simulink model "mcb_microchip_pmsm_foc_sensorless_dsPIC33EP256MC506"  (R2024b)
settings: Solver=FixedStepDiscrete  StartTime=0.0  StopTime=10  FixedStep=Ts  RelTol=1e-3  EnableMultiTasking=on
InitFcn:
  | mcb_microchip_pmsm_foc_sensorless_dsPIC33_data;
undefined symbols (not defined in the file): A4, C5, D8, F1, inverter, P20, P53, P97, PI_params, Pin, pmsm, PU_System, PWM_frequency, PWMmax, Speed_openLoop_PU, Ts, Ts_speed
libraries: MCHP_Blockset x16, mcbcontrolslib x10, simulink x9, slpidlib x3, mcbpositiondecoderlib x2, mcbplantlib x1, autolibpmsmexterior x1
(part 2 of 3)

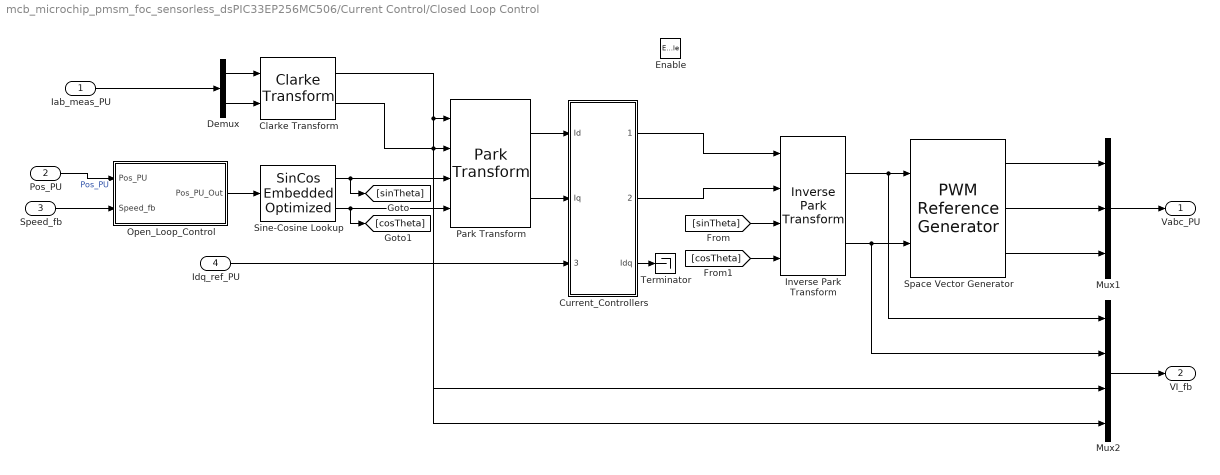
== system mcb_microchip_pmsm_foc_sensorless_dsPIC33EP256MC506/Current Control/Closed Loop Control ==
  Iab_meas_PU : Inport
  Pos_PU : Inport  Port=2
  Speed_fb : Inport  Port=3
  Idq_ref_PU : Inport  Port=4
  Enable : EnablePort
  Clarke Transform : mcbcontrolslib/Clarke Transform  VariantControl=Variant2  PhaseInput=Two inputs  EnPowerInv=off
  Current_Controllers : Subsystem
  Demux : Demux  Outputs=2
  Inverse Park Transform : mcbcontrolslib/Inverse Park Transform  PhaseInput=Two inputs  AxisAlignment=D-axis  ThetaInput=Sine and Cosine electrical position  AngleInput=Per-unit  N_points=1024
  Mux1 : Mux  Inputs=3
  Mux2 : Mux
  Open_Loop_Control : Subsystem
  Park Transform : mcbcontrolslib/Park Transform  PhaseInput=Two inputs  AxisAlignment=D-axis  ThetaInput=Sine and Cosine electrical position  AngleInput=Per-unit  N_points=1024
  Sine-Cosine Lookup : mcbcontrolslib/SinCos Embedded Optimized  LabelModeActiveChoice=MCB_Sin  OptforProc=off  ApproximationMethod=None  UserApproxMethod=Lookup  ApproxStatus=None  InterpMethod=Linear point-slope  NumberOfDataPoints=16  NumberOfIterations=11  RemoveProtectionAgainstOutOfRangeInput=off  TableDataTypeStr=Inherit: Inherit via input  AngleInput=Per-unit  ThetaDataType=single  N_points=1024  DatatypeInput=Inherit from input  Datatype=Inherit: Same as input
  Space Vector Generator : mcbcontrolslib/PWM Reference Generator  inSignal=Valphabeta  modType=SVM: space vector modulation
  Terminator : Terminator
  Vabc_PU : Outport  OutputWhenDisabled=reset  InitialOutput=[0 0 0]  VectorParamsAs1DForOutWhenUnconnected=off
  VI_fb : Outport  Port=2  OutputWhenDisabled=reset  InitialOutput=[0 0 0 0]  VectorParamsAs1DForOutWhenUnconnected=off
  wires:
  Current_Controllers/1(Vd_ref) -> Inverse Park Transform/1
  [sinTheta] -> Inverse Park Transform/3
  Sine-Cosine Lookup/1 -> [sinTheta], Park Transform/3
  Space Vector Generator/1 -> Mux1/1
  Space Vector Generator/3 -> Mux1/3
  Sine-Cosine Lookup/2 -> Park Transform/4, [cosTheta]
  Space Vector Generator/2 -> Mux1/2
  Idq_ref_PU/1 -> Current_Controllers/3(Idq_ref_PU)
  Iab_meas_PU/1 -> Demux/1
  Demux/1 -> Clarke Transform/1
  Demux/2 -> Clarke Transform/2
  Park Transform/2 -> Current_Controllers/2(Iq)
  [cosTheta] -> Inverse Park Transform/4
  Current_Controllers/2(Vq_ref) -> Inverse Park Transform/2
  Mux1/1 -> Vabc_PU/1
  Speed_fb/1 -> Open_Loop_Control/2(Speed_fb)
  Current_Controllers/3(Idq) -> Terminator/1
  Park Transform/1 -> Current_Controllers/1(Id)
  Pos_PU/1 -> Open_Loop_Control/1(Pos_PU)  "Pos_PU"
  Open_Loop_Control/1(Pos_PU_Out) -> Sine-Cosine Lookup/1
  Mux2/1 -> VI_fb/1
  Inverse Park Transform/1 -> Mux2/1, Space Vector Generator/1
  Clarke Transform/2 -> Mux2/4, Park Transform/2
  Inverse Park Transform/2 -> Space Vector Generator/2, Mux2/2
  Clarke Transform/1 -> Mux2/3, Park Transform/1

== system mcb_microchip_pmsm_foc_sensorless_dsPIC33EP256MC506/Current Control/Input Scaling ==
  Iab_PU_In : Inport
  Iab_PU_Sim : Inport  Port=2
  VI_fb : Inport  Port=3
  DC component removal : Subsystem
  Sensorless : Subsystem
  Variant Source : VariantSource
  Iab_PU : Outport
  Pos_PU : Outport  Port=2
  Speed_meas_PU : Outport  Port=3
  tag scope: Speed=global
  wires:
  Iab_PU_Sim/1 -> Variant Source/2
  Variant Source/1 -> Iab_PU/1
  DC component removal/1(SigOUT) -> Sensorless/1(VI_fb)
  VI_fb/1 -> DC component removal/1(SigIN)  "Pos"
  Sensorless/2(Theta) -> Pos_PU/1  "Pos"
  Sensorless/1(Speed_meas_PU) -> [Speed], Speed_meas_PU/1
  Iab_PU_In/1 -> Variant Source/1

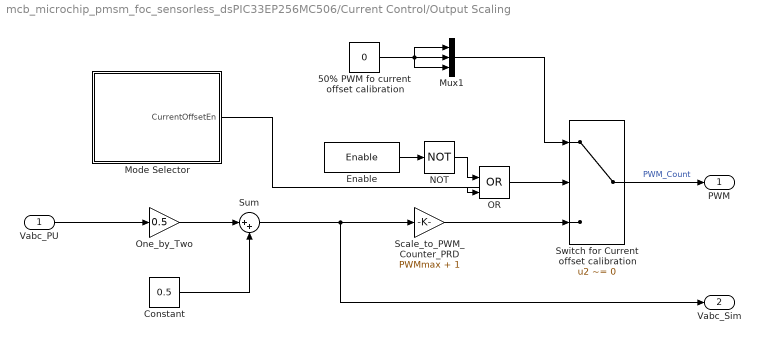
== system mcb_microchip_pmsm_foc_sensorless_dsPIC33EP256MC506/Current Control/Output Scaling ==
  Vabc_PU : Inport
  50% PWM fo current offset calibration : Constant  Value=0  OutDataTypeStr=Inherit: Inherit via back propagation
  Constant : Constant  Value=0.5  OutDataTypeStr=dataType  SampleTime=-1
  Enable : DataStoreRead  DataStoreName=Enable  IndexOptions=Index vector (dialog)  Indices=1  OutputSizes=1
  Mode Selector : Subsystem
  Mux1 : Mux  Inputs=3
  NOT : Logic  Operator=NOT  IconShape=distinctive  AllPortsSameDT=off  OutDataTypeStr=boolean
  OR : Logic  Operator=OR  IconShape=distinctive  AllPortsSameDT=off  OutDataTypeStr=boolean
  One_by_Two : Gain  Gain=0.5  RndMeth=Simplest  OutDataTypeStr=Inherit: Same as input
  Scale_to_PWM_Counter_PRD : Gain  Gain=PWMmax + 1  OutDataTypeStr=uint16  RndMeth=Simplest
  Sum : Sum  Inputs=|++
  Switch for Current offset calibration : Switch  Criteria=u2 ~= 0  Threshold=250  SaturateOnIntegerOverflow=off  InputSameDT=off
  PWM : Outport
  Vabc_Sim : Outport  Port=2
  wires:
  Constant/1 -> Sum/2
  One_by_Two/1 -> Sum/1
  Vabc_PU/1 -> One_by_Two/1
  Mux1/1 -> Switch for Current offset calibration/1
  50% PWM fo current offset calibration/1 -> Mux1/1, Mux1/3, Mux1/2
  Mode Selector/1(CurrentOffsetEn) -> OR/2
  OR/1 -> Switch for Current offset calibration/2
  Enable/1 -> NOT/1
  NOT/1 -> OR/1
  Scale_to_PWM_Counter_PRD/1 -> Switch for Current offset calibration/3
  Sum/1 -> Vabc_Sim/1, Scale_to_PWM_Counter_PRD/1
  Switch for Current offset calibration/1 -> PWM/1  "PWM_Count"

== system mcb_microchip_pmsm_foc_sensorless_dsPIC33EP256MC506/Current Control/PWM Driver ==
  PWM (abc) : Inport
  Dead time Compensation : Bias  Bias=round( (inverter.deadtime/Ts) *PWMmax )  SaturateOnIntegerOverflow=off
  Demux : Demux  Outputs=3
  PWM High Speed : MCHP_Blockset/PWM IO/PWM High Speed  pop1=[1]  chk1="[1  1  1  0  0]"  chkHL1="[1  1  1  1  1  1  1  1 ; 1  1  1  1  1  1  1  1]"  maxP1={ 'Ts','5e-05','5e-05','0.001','0.001','0.001','0.001','0.001';'0.001','0.001','1e-06','0.001','0.001','0.001','0.001','0.001'}  InitP2={ 'Ts','5e-05','5e-05','0.001','0.001','0.001','0.001','0.001';'0.001','0.001','0.001','0.001','0.001','0.001','0.001','0.001'}  chkP2="[0  0  0  1  1  1  1  1 ; 1  0  0  1  1  1  1  1]"  InitDC={ '4','4','4','50','50','50','50','50';'0.001','0.001','0.001','50','50','50','50','50'}  chkDC="[1  1  1  1  1  1  1  1 ; 0  0  0  1  1  1  1  1]"  InitPh={ '0','0','0','0.001','0.001','0.001','0.001','0.001';'0','0','0','0.001','0.001','0.001','0.001','0.001'}  chkPh="[0  0  0  1  1  1  1  1 ; 0  0  0  1  1  1  1  1]"  edSEvTrigx={ '0','-1','-1','-1','-1','-1','-1','-1'}  chkSEvTrigx="[0  0  0  1  1  1  1  1]"  popFlt="[2  2  2  1  1  1  1  1]"  popFltPin="[20  20  20   4   4   4   4   4]"  popFltPinRp="[1  1  1  1  1  1  1]"  popFltActivH="[2  2  2  1  1  1  1  1]"  popFltForceH="[2  2  2  2  2  2  2  2]"  popFltForceL="[1  1  1  1  1  1  1  1]"  chkFltBlkOut="[0  0  0  0  0  0  0  0]"  popIndepFaultMode="[1  1  1  1  1  1  1  1]"  popCurEnabled="[1  1  1  1  1  1  1  1]"  popCurPin="[4  31   4   4   4   4   4   4]"  popCurActiveH="[1  1  1  1  1  1  1  1]"  popCurForceH="[2  1  2  1  1  1  1  1]"  popCurForceL="[2  1  2  1  1  1  1  1]"  ChkCurBlkOut="[1  0  0  0  0  0  0  0]"  ChkCurBlkOutTime="[1  0  1  0  0  0  0  0]"  popBLANKSEL="[1  1  1  1  1  1  1  1]"  popBPHHBPHL="[1  1  1  1  1  1  1  1]"  popBPLHBPLL="[1  1  1  1  1  1  1  1]"  popFLTLEBEN_CLLEBEN="[1  1  1  1  1  1  1  1]"  popPHR_PHF="[2  1  1  1  1  1  1  1]"  popPLR_PLF="[3  1  1  1  1  1  1  1]"  edLEB={ '100e-9','50e-9','150e-9','50e-9','50e-9','50e-9','50e-9','50e-9'}  popDT="[1  1  1  3  3  3  3  3]"  edDTRx={ '0','0','0','1e-05','1e-05','1e-05','1e-05','1e-05'}  edAltDTRx={ 'inverter.deadtime','inverter.deadtime','inverter.deadtime','1e-05','1e-05','1e-05','1e-05','1e-05'}  S_INPUT="[5  5  5]"  S_INPUT_Size="[1  1  1]"  S_OUTPUT=[]  S_OUTPUT_Size=[]  S_DWORK_Type=[]  S_DWORK_Size=[]  ADC_VARTRIG={PWM Primary Special Event Trigger;6}  evalin_ws=PWMmax = 3499;PWM1max = 3499;PWM2max = 3499;PWM3max = 3499;  SampleTime=-1  ORDERING=None  MCHP_PORT={PWM1 Fault}{FLT32}4:0:B4;{PWM2 Fault}{FLT32}4:0:B4;{PWM3 Fault}{FLT32}4:0:B4;{PWM1H}{PWM1H}4:4:B14;{PWM1L}{PWM1L}4:4:B15;{PWM2H}{PWM2H}4:4:B12;{PWM2L}{PWM2L}4:4:B13;{PWM3H}{PWM3H}4:4:B10;{PWM3L}{PWM3L}4:4:B11;  MCHP_MASTERLINK=mcb_microchip_pmsm_foc_sensorless_dsPIC33EP256MC506/Hardware Init/Microchip Master  MCHP_VERSION=v3.38  Parameter50=0
      settings: SourceProductName=MPLAB Device Blocks for Simulink
  Saturation low side turn on errate workaround + errata for Phase shift (times 2) : Saturate  UpperLimit=PWMmax  LowerLimit=round( (inverter.deadtime/Ts) *PWMmax )* 2
  int to uint : DataTypeConversion  OutDataTypeStr=uint16  ConvertRealWorld=Stored Integer (SI)  SaturateOnIntegerOverflow=off  RndMeth=Floor
  wires:
  int to uint/1 -> Saturation low side turn on errate workaround + errata for Phase shift (times 2)/1
  Dead time Compensation/1 -> int to uint/1
  PWM (abc)/1 -> Dead time Compensation/1
  Saturation low side turn on errate workaround + errata for Phase shift (times 2)/1 -> Demux/1
  Demux/1 -> PWM High Speed/1
  Demux/2 -> PWM High Speed/2
  Demux/3 -> PWM High Speed/3

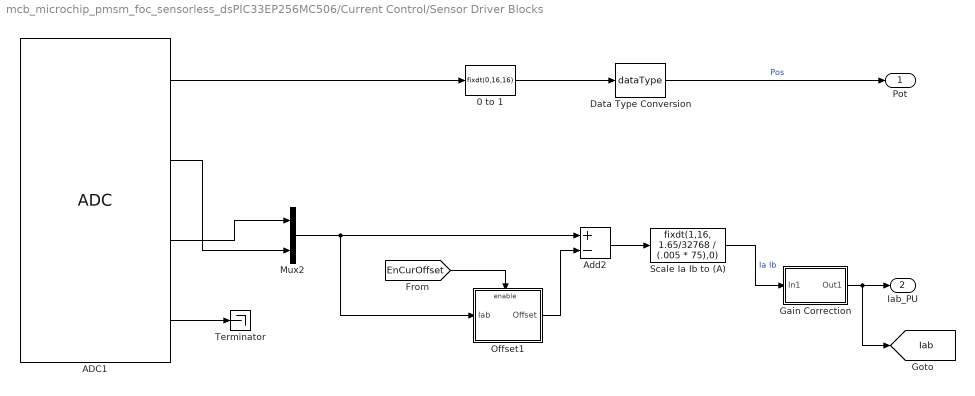
== system mcb_microchip_pmsm_foc_sensorless_dsPIC33EP256MC506/Current Control/Sensor Driver Blocks ==
  0 to 1 : DataTypeConversion  OutDataTypeStr=fixdt(0,16,16)  ConvertRealWorld=Stored Integer (SI)  SaturateOnIntegerOverflow=off  RndMeth=Floor
  ADC1 : MCHP_Blockset/Analog IO/ADC  Priority=5  ADC_REF=1  Mode=10 bits (allows exact simultaneous sampling)  FORM=dddd dddd dddd 0000 ==> Unsigned fractional  ADC_R="< 5    kOhm"  nSAMPLECHANNELS=CH0 : CH1 : CH2 : CH3  nSAMPLECHANNELS_12bits=CH0 only  SIMULTANEOUS=Simultaneously on all Channels  ADxCSS=[13]  MUXA_CH0N=off  MUXA_CH123_TXT=AN0 : AN1 : AN2  MUXB_CH0=AN13  MUXB_CH0N=on  MUXB_CH123_TXT=AN0 : AN1 : AN2  SequenceRepeat=1  SequenceTiming=are done as fast as possible ; triggered by user define source  SSRC_SSRCG_TXT=6  Update_BlockOutput=After each trig and conversion sequence  Trig_TimeStep=with each update of the ADC block output  ADC_DMA_CHANNEL=Use Interrupt instead of DMA  SampleTime=5e-05  Info=Total Time for Sample & Conversion : 4.4571e-06s including 3.4286e-07s (x 1) sample time.  MCHP_PORT={Analog Input 0}{AN0}15:2:A0;{Analog Input 1}{AN1}15:2:A1;{Analog Input 2}{AN2}15:2:B0;{Analog Input 13}{AN13}15:2:E13;  MCHP_MASTERLINK=mcb_microchip_pmsm_foc_sensorless_dsPIC33EP256MC506/Hardware Init/Microchip Master  ADC_TIMING=[4.4571428571428571832e-06]
      settings: SourceProductName=MPLAB Device Blocks for Simulink
  Add2 : Sum  Inputs=+-  OutDataTypeStr=int16  RndMeth=Zero
  Data Type Conversion : DataTypeConversion  OutDataTypeStr=dataType  RndMeth=Simplest  SaturateOnIntegerOverflow=off
  Gain Correction : Subsystem
  Mux2 : Mux  Inputs=2
  Offset1 : Subsystem
  Scale Ia Ib to (A) : DataTypeConversion  OutDataTypeStr=fixdt(1,16, 1.65/32768 / (.005 * 75),0)  ConvertRealWorld=Stored Integer (SI)  SaturateOnIntegerOverflow=off
  Terminator : Terminator
  Pot : Outport  VectorParamsAs1DForOutWhenUnconnected=off
  Iab_PU : Outport  Port=2  VectorParamsAs1DForOutWhenUnconnected=off
  tag scope: Iab=global
  wires:
  Mux2/1 -> Offset1/1(Iab), Add2/1
  0 to 1/1 -> Data Type Conversion/1
  [EnCurOffset] -> Offset1/Enable
  Data Type Conversion/1 -> Pot/1  "Pos"
  Add2/1 -> Scale Ia Ib to (A)/1
  ADC1/3 -> Mux2/1
  ADC1/1 -> 0 to 1/1
  Offset1/1(Offset) -> Add2/2
  ADC1/2 -> Mux2/2
  ADC1/4 -> Terminator/1
  Scale Ia Ib to (A)/1 -> Gain Correction/1(In1)  "Ia Ib"
  Gain Correction/1(Out1) -> [Iab], Iab_PU/1

== system mcb_microchip_pmsm_foc_sensorless_dsPIC33EP256MC506/Current Control/To Matlab Host  ==
  note: Note: Uncomment above blocks and comment Serial Send (below) to use Microchip's picgui interface to log hardware signals
  speed : Inport
  Data Store Read2 : DataStoreRead  DataStoreName=Speed_ref  IndexOptions=Index vector (dialog)  Indices=1  OutputSizes=1
  Gain : Gain  Gain=PU_System.N_base  OutDataTypeStr=uint16  RndMeth=Simplest
  Gain1 : Gain  Gain=PU_System.N_base  OutDataTypeStr=uint16
  Serial Send : Subsystem
  UART Tx-Matlab : MCHP_Blockset/BUS UART/UART Tx-Matlab  Commented=on  UART_REF=2  CHANNELS=[1 2]  AllOrNothing=off  SampleTime=.001  MCHP_MASTERLINK=mcb_microchip_pmsm_foc_sensorless_dsPIC33EP256MC506/Hardware Init/Microchip Master  MCHP_COMPILED_INFO="CompiledSampleTime= [0.0010000000000000000208   0 ];CompiledInportDataTypes=[  4   4 ];CompiledInportDataWidth=[1  1];"
      settings: SourceProductName=MPLAB Device Blocks for Simulink
  int to uint2 : DataTypeConversion  OutDataTypeStr=int16  ConvertRealWorld=Stored Integer (SI)  SaturateOnIntegerOverflow=off  RndMeth=Floor
  int to uint3 : DataTypeConversion  OutDataTypeStr=int16  ConvertRealWorld=Stored Integer (SI)  SaturateOnIntegerOverflow=off  RndMeth=Floor
  picgui Graphical interface : MCHP_Blockset/BUS UART/picgui Graphical interface  Commented=on  Nothing=0
      settings: SourceProductName=MPLAB Device Blocks for Simulink
  wires:
  speed/1 -> Serial Send/2(Speed_fb), Gain1/1
  Data Store Read2/1 -> Serial Send/1(Speed_ref), Gain/1
  Gain/1 -> int to uint3/1
  Gain1/1 -> int to uint2/1
  int to uint3/1 -> UART Tx-Matlab/1  "U2 CH1"
  int to uint2/1 -> UART Tx-Matlab/2  "U2 CH2"

== system mcb_microchip_pmsm_foc_sensorless_dsPIC33EP256MC506/Hardware Init/Open Board and Motor pages ==

== system mcb_microchip_pmsm_foc_sensorless_dsPIC33EP256MC506/Inverter and Motor/Codegeneration ==
  Duty_Cycles : Inport
  Ground : Ground
  Terminator : Terminator
  Feedbacks_Iab : Outport  VectorParamsAs1DForOutWhenUnconnected=off
  wires:
  Ground/1 -> Feedbacks_Iab/1
  Duty_Cycles/1 -> Terminator/1

== system mcb_microchip_pmsm_foc_sensorless_dsPIC33EP256MC506/Inverter and Motor/Simulation ==
  Duty_Cycles : Inport
  Inverter : Subsystem
  Load_Profile (Torque) : Subsystem
  Sensor_Measurements : Subsystem
  Surface Mount PMSM : autolibpmsmexterior/Surface Mount PMSM  port_config=Torque  sim_type=Discrete  Ts=Ts  P=pmsm.p  Rs=pmsm.Rs + inverter.R_board  Ldq_=pmsm.Ld  KConstText=Permanent flux linkage constant (lambda_pm):  lambda_pm=pmsm.FluxPM  Ke=159.9771  Kt=1.323  mechanical=[pmsm.J, pmsm.B, 0]  idq0=[0 0]  theta_init=0  omega_init=0  KConst=pmsm.FluxPM  lambda_pm_calc=pmsm.FluxPM  RefBlkName='autolibpmsmexterior/Surface Mount PMSM'  aMode=5  Ldq="[0.0002      0.0002]"
  Terminator : Terminator
  Terminator1 : Terminator
  Feedbacks_Iab : Outport  VectorParamsAs1DForOutWhenUnconnected=off
  wires:
  Surface Mount PMSM/3 -> Terminator/1
  Duty_Cycles/1 -> Inverter/1(Duty_abc)
  Surface Mount PMSM/2 -> Sensor_Measurements/1(PhaseCurr)  "Iabc"
  Sensor_Measurements/1(Iab_fb) -> Feedbacks_Iab/1
  Load_Profile (Torque)/1(Load_Trq) -> Surface Mount PMSM/1
  Inverter/1(Vabc) -> Surface Mount PMSM/2
  Surface Mount PMSM/1 -> Terminator1/1

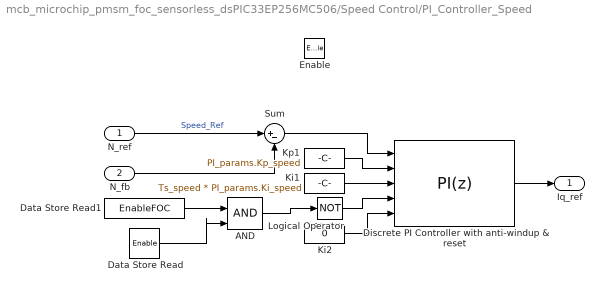
== system mcb_microchip_pmsm_foc_sensorless_dsPIC33EP256MC506/Speed Control/PI_Controller_Speed ==
  N_ref : Inport
  N_fb : Inport  Port=2
  Enable : EnablePort
  AND : Logic  IconShape=distinctive  AllPortsSameDT=off  OutDataTypeStr=boolean
  Data Store Read : DataStoreRead  DataStoreName=Enable  IndexOptions=Index vector (dialog)  Indices=1  OutputSizes=1
  Data Store Read1 : DataStoreRead  DataStoreName=EnableFOC  IndexOptions=Index vector (dialog)  Indices=1  OutputSizes=1
  Discrete PI Controller with anti-windup & reset : slpidlib/PID Controller  Controller=PI  Form=Parallel  TimeDomain=Discrete-time  UseExternalTs=off  SampleTime=-1  IntegratorMethod=Forward Euler  FilterMethod=Forward Euler  ControllerParametersSource=external  P=1  I=1  UseKiTs=on  D=0  UseExternalDerivativeSource=off  N=100  UseFilter=on  TunerSelectOption=Transfer Function Based (PID Tuner App)  InitialConditionSource=external  InitialConditionForIntegrator=0  InitialConditionForFilter=0  DifferentiatorICPrevScaledInput=0  ExternalReset=level  TrackingMode=off  Kt=1  LimitOutput=on  SatLimitsSource=internal  UpperSaturationLimit=1  LowerSaturationLimit=-1  LinearizeAsGain=on  AntiWindupMode=clamping  Kb=1  LimitIntegrator=off  UpperIntegratorSaturationLimit=inf  LowerIntegratorSaturationLimit=-inf  RndMeth=Simplest  POutMin=[]  POutMax=[]  IOutMin=[]  IOutMax=[]  DOutMin=[]  DOutMax=[]  NOutMin=[]  NOutMax=[]  SumOutMin=[]  SumOutMax=[]  SaturationOutDataTypeStr=Inherit: Inherit via back propagation  SaturationOutMin=[]  SaturationOutMax=[]  PParamMin=[]  PParamMax=[]  IParamMin=[]  IParamMax=[]  DParamMin=[]  DParamMax=[]  NParamMin=[]  NParamMax=[]  KbParamMin=[]  KbParamMax=[]  KtParamMin=[]  KtParamMax=[]  KbOutMin=[]  KbOutMax=[]  KtOutMin=[]  KtOutMax=[]  IntegratorOutMin=[]  IntegratorOutMax=[]  FilterOutMin=[]  FilterOutMax=[]  SumI1OutMin=[]  SumI1OutMax=[]  SumI2OutMin=[]  SumI2OutMax=[]  SumI3OutMin=[]  SumI3OutMax=[]  SumI4OutMin=[]  SumI4OutMax=[]  SumDOutMin=[]  SumDOutMax=[]  DifferentiatorOutMin=[]  DifferentiatorOutMax=[]  FilterDiffOutCoefMin=[]  FilterDiffOutCoefMax=[]  ReciprocalOutMin=[]  ReciprocalOutMax=[]  SumDenOutMin=[]  SumDenOutMax=[]  SumNumOutMin=[]  SumNumOutMax=[]  DivideOutMin=[]  DivideOutMax=[]  UdiffTsProdOutMin=[]  UdiffTsProdOutMax=[]  NTsProdOutMin=[]  NTsProdOutMax=[]  UintegralTsProdOutMin=[]  UintegralTsProdOutMax=[]  UngainTsProdOutMin=[]  UngainTsProdOutMax=[]  ClampingZeroOutDataTypeStr=Inherit: Inherit via back propagation  ClampingZeroOutMin=[]  ClampingZeroOutMax=[]  FilterDenConstantOutDataTypeStr=Inherit: Inherit via back propagation  FilterDenConstantOutMin=[]  FilterDenConstantOutMax=[]  PCopyOutDataTypeStr=Inherit: Inherit via back propagation  PCopyOutMin=[]  PCopyOutMax=[]  NCopyOutDataTypeStr=Inherit: Inherit via back propagation  NCopyOutMin=[]  NCopyOutMax=[]  IntegratorContinuousStateAttributes=''  IntegratorStateMustResolveToSignalObject=off  IntegratorRTWStateStorageClass=Auto  FilterContinuousStateAttributes=''  FilterStateMustResolveToSignalObject=off  FilterRTWStateStorageClass=Auto  ParallelPVariant=ExternalParameters  IdealPVariant=Disabled  IVariant=ExternalParameters  DVariant=Disabled  IntegratorVariant=Discrete  SatVariant=Enabled  AWVariant=DiscClampingParallel  PCopyVariant=Disabled  TRVariant=Disabled  FdbkBlocksVariant=Forward  IdealPFdbkVariant=Disabled  SatFdbkVariant=Disabled  DerivativeFilterVariant=Disabled  NVariant=Disabled  NCopyVariant=Disabled_SignalSpec  FilterICVariant=Disabled  IntegratorICVariant=ExternalICs  ExternalResetVariant=ExternalReset  TRSumVariant=Passthrough  SumFdbkVariant=Disabled  SumVariant=Sum_PI  TsampFilterVariant=InternalTs  TsampNgainVariant=Passthrough  TsampIntegralVariant=Disabled_SignalSpec  ExternalSaturationOutDataTypeStr=Inherit: Same as second input  DerivativeSourceVariant=Disabled  PreIntVariant=InternalPreInt
      settings: LibrarySourceBlock=mcbcontrolslib/PI Controller
  Ki1 : Constant  Value=Ts_speed * PI_params.Ki_speed  OutDataTypeStr=dataType  SampleTime=-1
  Ki2 : Constant  Value=0  OutDataTypeStr=dataType  SampleTime=-1
  Kp1 : Constant  Value=PI_params.Kp_speed  OutDataTypeStr=dataType2  SampleTime=-1
  Logical Operator : Logic  Operator=NOT  IconShape=distinctive  AllPortsSameDT=off  OutDataTypeStr=boolean
  Sum : Sum  Inputs=|+-  OutDataTypeStr=Inherit: Same as first input
  Iq_ref : Outport  OutputWhenDisabled=reset  InitialOutput=0  VectorParamsAs1DForOutWhenUnconnected=off
  wires:
  Discrete PI Controller with anti-windup & reset/1 -> Iq_ref/1
  Ki1/1 -> Discrete PI Controller with anti-windup & reset/3
  Kp1/1 -> Discrete PI Controller with anti-windup & reset/2
  N_fb/1 -> Sum/2
  Sum/1 -> Discrete PI Controller with anti-windup & reset/1
  Logical Operator/1 -> Discrete PI Controller with anti-windup & reset/4
  Ki2/1 -> Discrete PI Controller with anti-windup & reset/5
  N_ref/1 -> Sum/1  "Speed_Ref"
  Data Store Read1/1 -> AND/1
  Data Store Read/1 -> AND/2
  AND/1 -> Logical Operator/1

== system mcb_microchip_pmsm_foc_sensorless_dsPIC33EP256MC506/Speed Control/Speed_Ref_Selector ==
  Speed_Ref : Inport
  Constant : Constant  Value=Speed_openLoop_PU  OutDataTypeStr=dataType
  Data Store Read1 : DataStoreRead  DataStoreName=EnClosedLoop  IndexOptions=Index vector (dialog)  Indices=1  OutputSizes=1
  Switch : Switch  Criteria=u2 > Threshold  SaturateOnIntegerOverflow=off  InputSameDT=off
  Zero_Cancellation : mcbcontrolslib/IIR Filter  VariantControl=Low Pass Filter  VariantSelect=Low-pass  FilterConstantInputType=Specify via dialog  Filter_constant=0.2  advancedSettings=off  Ts=50e-6  cutOff_freq=795.7747
  Speed_ref : Outport
  wires:
  Constant/1 -> Switch/3
  Data Store Read1/1 -> Switch/2
  Switch/1 -> Zero_Cancellation/1
  Speed_Ref/1 -> Switch/1
  Zero_Cancellation/1 -> Speed_ref/1

== system mcb_microchip_pmsm_foc_sensorless_dsPIC33EP256MC506/System Inputs/Adjust Pot output ==
  note: Toggle between enable and disable on press on Button S2
  In1 : Inport
  Add : Sum
  Button S2 : MCHP_Blockset/Digital IO/Digital Input  PORT_TXT="G   [ 6 : 9 ]"  PIN=7  INPUT_PIN_MODE=Hi-impedance (default)  PACK=off  SIMULTANEOUS=off  ORDERING=None  SampleTime=-1  MCHP_PORT={Digital In}{DIN}2:0:G7;  MCHP_MASTERLINK=mcb_microchip_pmsm_foc_sensorless_dsPIC33EP256MC506/Hardware Init/Microchip Master
      settings: SourceProductName=MPLAB Device Blocks for Simulink
  Constant : Constant  Value=0.3
  Gain : Gain  Gain=0.45
  Saturation : Saturate  UpperLimit=0.75  LowerLimit=0.3
  Triggered Subsystem : Subsystem  TreatAsAtomicUnit=on
  Out1 : Outport
  wires:
  In1/1 -> Gain/1
  Constant/1 -> Add/2
  Gain/1 -> Add/1
  Add/1 -> Saturation/1
  Saturation/1 -> Out1/1
  Button S2/1 -> Triggered Subsystem/Trigger

== system mcb_microchip_pmsm_foc_sensorless_dsPIC33EP256MC506/System Inputs/Sim ==
  Data Store Write : DataStoreWrite  DataStoreName=Enable  IndexOptions=Index vector (dialog)  Indices=1  OutputSizes=1
  Data Type Conversion : DataTypeConversion  SaturateOnIntegerOverflow=off  RndMeth=Floor
  Enable : Step  Time=0.5  SampleTime=0
  Speed Ref (Sim) : Step  Time=4  Before=0.5  After=0.75  OutDataTypeStr=Inherit: Inherit via back propagation
  Out1 : Outport
  wires:
  Speed Ref (Sim)/1 -> Out1/1
  Data Type Conversion/1 -> Data Store Write/1
  Enable/1 -> Data Type Conversion/1

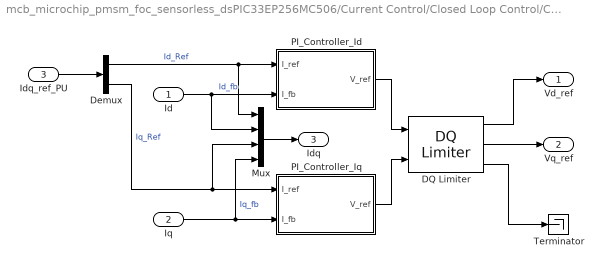
== system mcb_microchip_pmsm_foc_sensorless_dsPIC33EP256MC506/Current Control/Closed Loop Control/Current_Controllers ==
  Id : Inport
  Iq : Inport  Port=2
  Idq_ref_PU : Inport  Port=3
  DQ Limiter : mcbcontrolslib/DQ Limiter  satMethodInputType=Specify via dialog  satMethodSelected=D-Q equivalence  satLimitInputType=Specify via dialog  Vmax=0.95
  Demux : Demux  Outputs=2
  Mux : Mux
  PI_Controller_Id : Subsystem
  PI_Controller_Iq : Subsystem
  Terminator : Terminator
  Vd_ref : Outport  VectorParamsAs1DForOutWhenUnconnected=off
  Vq_ref : Outport  Port=2  VectorParamsAs1DForOutWhenUnconnected=off
  Idq : Outport  Port=3  VectorParamsAs1DForOutWhenUnconnected=off
  wires:
  Iq/1 -> Mux/4, PI_Controller_Iq/2(I_fb)  "Iq_fb"
  Id/1 -> Mux/2, PI_Controller_Id/2(I_fb)  "Id_fb"
  Demux/1 -> Mux/1, PI_Controller_Id/1(I_ref)  "Id_Ref"
  Demux/2 -> Mux/3, PI_Controller_Iq/1(I_ref)  "Iq_Ref"
  Idq_ref_PU/1 -> Demux/1
  DQ Limiter/3 -> Terminator/1
  Mux/1 -> Idq/1
  PI_Controller_Iq/1(V_ref) -> DQ Limiter/2
  PI_Controller_Id/1(V_ref) -> DQ Limiter/1
  DQ Limiter/1 -> Vd_ref/1
  DQ Limiter/2 -> Vq_ref/1

== system mcb_microchip_pmsm_foc_sensorless_dsPIC33EP256MC506/Current Control/Closed Loop Control/Open_Loop_Control ==
  Pos_PU : Inport
  Speed_fb : Inport  Port=2
  Constant : Constant  Value=Speed_openLoop_PU  OutDataTypeStr=dataType
  Gain : Gain  Gain=Ts*PU_System.N_base*pmsm.p/60  OutDataTypeStr=Inherit: Same as input  ParamDataTypeStr=Inherit: Same as input
  OpentoClosed : Subsystem
  Position Generator : mcbcontrolslib/Position Generator  AngleOutput=Per-unit  ExternalReset=none  Offset=0
  Switch : Switch  Criteria=u2 ~= 0  SaturateOnIntegerOverflow=off  InputSameDT=off
  Pos_PU_Out : Outport
  wires:
  Position Generator/1 -> Switch/3  "Eps"
  Gain/1 -> Position Generator/1
  Switch/1 -> Pos_PU_Out/1
  Pos_PU/1 -> Switch/1
  Constant/1 -> Gain/1
  Speed_fb/1 -> OpentoClosed/1(Speed_fb)
  OpentoClosed/1(EnClosedLoop) -> Switch/2

== system mcb_microchip_pmsm_foc_sensorless_dsPIC33EP256MC506/Current Control/Input Scaling/DC component removal ==
  SigIN : Inport
  Data Type Conversion1 : DataTypeConversion  OutDataTypeStr=dataType  SaturateOnIntegerOverflow=off
  High Pass Filter 1 : Subsystem  Tag=FilterWizardSubSystem
  SigOUT : Outport
  wires:
  SigIN/1 -> High Pass Filter 1/1(Input)
  High Pass Filter 1/1(Output) -> Data Type Conversion1/1
  Data Type Conversion1/1 -> SigOUT/1

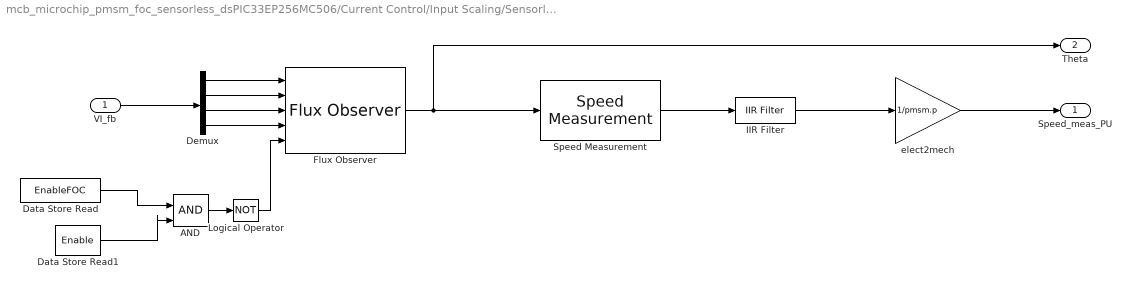
== system mcb_microchip_pmsm_foc_sensorless_dsPIC33EP256MC506/Current Control/Input Scaling/Sensorless ==
  VI_fb : Inport
  AND : Logic  IconShape=distinctive  AllPortsSameDT=off  OutDataTypeStr=boolean
  Data Store Read : DataStoreRead  DataStoreName=EnableFOC  IndexOptions=Index vector (dialog)  Indices=1  OutputSizes=1
  Data Store Read1 : DataStoreRead  DataStoreName=Enable  IndexOptions=Index vector (dialog)  Indices=1  OutputSizes=1
  Demux : Demux
  Flux Observer : mcbpositiondecoderlib/Flux Observer  MotorSelection=PMSM  DataTypeSelect=on  BlockInputUnit=Per-unit  PerUnitVoltage=PU_System.V_base  PerUnitCurrent=PU_System.I_base  PositionSelect=on  FluxSelect=off  TorqueSelect=off  PolePairs=4  StatorResistance=pmsm.Rs  StatorDAxisInductance=pmsm.Ld  StatorLeakageInductance=0.0068  RotorLeakageInductance=0.0068  MagnetizingInductance=0.0300  CutoffFreq=10  BlockSampleTime=Ts  ParameterBusInput=off  PositionUnit=Per-unit  PositionDatatype=dataType  FluxUnit=Weber  PerUnitFlux=0.1  FluxDatatype=single  TorqueUnit=Nm  PerUnitTorque=100  TorqueDatatype=single  DataType=1
      settings: LibrarySourceBlock=mcblib/Sensorless Estimators/Flux Observer
  IIR Filter : mcbcontrolslib/IIR Filter  VariantControl=Low Pass Filter  VariantSelect=Low-pass  FilterConstantInputType=Specify via dialog  Filter_constant=0.02  advancedSettings=off  Ts=50e-6  cutOff_freq=64.9612
  Logical Operator : Logic  Operator=NOT  IconShape=distinctive  AllPortsSameDT=off  OutDataTypeStr=boolean
  Speed Measurement : mcbpositiondecoderlib/Speed Measurement  PositionUnit=Per unit  PositionScalingDatatype=uint16  SpeedCalculationMode=Time interval for speed calculation  SampleTimeAsync=Ts  MaximumApplicationSpeed=1000  SpeedResolution=5e-6  DelayLength=20  MaximumMeasurableSpeed=29999  MeasurableSpeedResolution=0.91553  SpeedUnit=Per unit based on dialog  PerUnitSpeed=PU_System.N_base  SpeedDataType=dataType2
      settings: LibrarySourceBlock=mcblib/Sensor Decoders/Speed Measurement
  elect2mech : Gain  Gain=1/pmsm.p  OutDataTypeStr=dataType  RndMeth=Simplest
  Speed_meas_PU : Outport
  Theta : Outport  Port=2
  wires:
  Demux/3 -> Flux Observer/3
  Demux/1 -> Flux Observer/1
  VI_fb/1 -> Demux/1
  Demux/4 -> Flux Observer/4
  Demux/2 -> Flux Observer/2
  IIR Filter/1 -> elect2mech/1
  elect2mech/1 -> Speed_meas_PU/1
  Speed Measurement/1 -> IIR Filter/1
  AND/1 -> Logical Operator/1
  Data Store Read/1 -> AND/1
  Data Store Read1/1 -> AND/2
  Flux Observer/1 -> Theta/1, Speed Measurement/1
  Logical Operator/1 -> Flux Observer/5

== system mcb_microchip_pmsm_foc_sensorless_dsPIC33EP256MC506/Current Control/Output Scaling/Mode Selector ==
  Delay : Delay  DelayLength=1
  NOT : Logic  Operator=NOT  IconShape=distinctive  AllPortsSameDT=off  OutDataTypeStr=boolean
  Subsystem1 : Subsystem
  Up Counter : Subsystem
  CurrentOffsetEn : Outport
  wires:
  Up Counter/1(Count) -> Subsystem1/1(Count)
  Delay/1 -> NOT/1
  NOT/1 -> Up Counter/Enable
  Subsystem1/2(EnClosedLoop) -> Delay/1
  Subsystem1/1(Current Offset) -> CurrentOffsetEn/1

== system mcb_microchip_pmsm_foc_sensorless_dsPIC33EP256MC506/Current Control/Sensor Driver Blocks/Gain Correction ==
  In1 : Inport
  Demux : Demux  Outputs=2
  Gain : Gain  Gain=0.9615  RndMeth=Zero  OutDataTypeStr=Inherit: Same as input
  Mux : Mux  Inputs=2
  To Per-Unit : Gain  Gain=inverter.invertingAmp/PU_System.I_base  OutMin=-1  OutMax=1  OutDataTypeStr=fixdt(1,16)  RndMeth=Zero
  Out1 : Outport
  wires:
  Demux/1 -> Gain/1
  Demux/2 -> Mux/2
  To Per-Unit/1 -> Demux/1
  Gain/1 -> Mux/1
  Mux/1 -> Out1/1
  In1/1 -> To Per-Unit/1

== system mcb_microchip_pmsm_foc_sensorless_dsPIC33EP256MC506/Current Control/Sensor Driver Blocks/Offset1 ==
  Iab : Inport
  Enable : EnablePort
  Offset : Outport
  wires:
  Iab/1 -> Offset/1

== system mcb_microchip_pmsm_foc_sensorless_dsPIC33EP256MC506/Current Control/To Matlab Host /Serial Send ==
  Speed_ref : Inport
  Speed_fb : Inport  Port=2
  Debug_Data : Subsystem
  SCI_Tx : Subsystem
  wires:
  Debug_Data/1(Data_log) -> SCI_Tx/1(Data_Log)
  Speed_fb/1 -> Debug_Data/2(In2)
  Speed_ref/1 -> Debug_Data/1(In1)

== system mcb_microchip_pmsm_foc_sensorless_dsPIC33EP256MC506/Inverter and Motor/Simulation/Inverter ==
  Duty_abc : Inport
  Average-Value Inverter : mcbplantlib/Average-Value Inverter
  Constant2 : Constant  Value=inverter.V_dc  OutDataTypeStr=single  SampleTime=-1
  Data Type Conversion1 : DataTypeConversion  OutDataTypeStr=single  RndMeth=Simplest  SaturateOnIntegerOverflow=off
  Vabc : Outport  VectorParamsAs1DForOutWhenUnconnected=off
  wires:
  Average-Value Inverter/1 -> Vabc/1
  Data Type Conversion1/1 -> Average-Value Inverter/1
  Duty_abc/1 -> Data Type Conversion1/1
  Constant2/1 -> Average-Value Inverter/2

== system mcb_microchip_pmsm_foc_sensorless_dsPIC33EP256MC506/Inverter and Motor/Simulation/Load_Profile (Torque) ==
  Data Type Conversion : DataTypeConversion  OutDataTypeStr=single  SaturateOnIntegerOverflow=off  RndMeth=Floor
  IIR Filter : mcbcontrolslib/IIR Filter  VariantControl=Low Pass Filter  VariantSelect=Low-pass  FilterConstantInputType=Specify via dialog  Filter_constant=0.0001  advancedSettings=off  Ts=50e-6  cutOff_freq=0.31834
  Step : Step  Time=2  After=0.2 * pmsm.T_rated
  Load_Trq : Outport  VectorParamsAs1DForOutWhenUnconnected=off
  wires:
  IIR Filter/1 -> Load_Trq/1
  Data Type Conversion/1 -> IIR Filter/1
  Step/1 -> Data Type Conversion/1

== system mcb_microchip_pmsm_foc_sensorless_dsPIC33EP256MC506/Inverter and Motor/Simulation/Sensor_Measurements ==
  note: Delays
  note: Scaling
  PhaseCurr : Inport
  Data Type Conversion4 : DataTypeConversion  OutDataTypeStr=single  RndMeth=Simplest  SaturateOnIntegerOverflow=off
  Delay1 : Delay  DelayLength=PI_params.delay_Currents
  Inverting OpAmp : Gain  Gain=1/PU_System.I_base  OutDataTypeStr=dataType  RndMeth=Simplest
  Selector : Selector  InputPortWidth=3  IndexOptions=Index vector (dialog)  Indices=[1 2]  OutputSizes=1
  Iab_fb : Outport  VectorParamsAs1DForOutWhenUnconnected=off
  wires:
  Selector/1 -> Inverting OpAmp/1
  PhaseCurr/1 -> Data Type Conversion4/1
  Data Type Conversion4/1 -> Delay1/1
  Delay1/1 -> Selector/1  "Iab_fb"
  Inverting OpAmp/1 -> Iab_fb/1

== system mcb_microchip_pmsm_foc_sensorless_dsPIC33EP256MC506/System Inputs/Adjust Pot output/Triggered Subsystem ==
  Trigger : TriggerPort  TriggerType=falling  VariantControl=Variant
  Data Store Write : DataStoreWrite  DataStoreName=Enable  IndexOptions=Index vector (dialog)  Indices=1  OutputSizes=1
  Delay : Delay  DelayLength=1  InitialCondition=0
  NOT : Logic  Operator=NOT  IconShape=distinctive  AllPortsSameDT=off  OutDataTypeStr=boolean
  wires:
  NOT/1 -> Data Store Write/1, Delay/1
  Delay/1 -> NOT/1

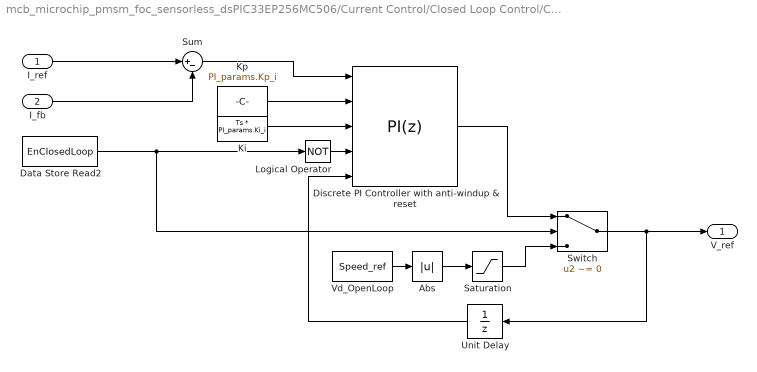
== system mcb_microchip_pmsm_foc_sensorless_dsPIC33EP256MC506/Current Control/Closed Loop Control/Current_Controllers/PI_Controller_Id ==
  I_ref : Inport
  I_fb : Inport  Port=2
  Abs : Abs  RndMeth=Simplest  SaturateOnIntegerOverflow=off
  Data Store Read2 : DataStoreRead  DataStoreName=EnClosedLoop  IndexOptions=Index vector (dialog)  Indices=1  OutputSizes=1
  Discrete PI Controller with anti-windup & reset : slpidlib/PID Controller  Controller=PI  Form=Parallel  TimeDomain=Discrete-time  UseExternalTs=off  SampleTime=-1  IntegratorMethod=Forward Euler  FilterMethod=Forward Euler  ControllerParametersSource=external  P=1  I=1  UseKiTs=on  D=0  UseExternalDerivativeSource=off  N=100  UseFilter=on  TunerSelectOption=Transfer Function Based (PID Tuner App)  InitialConditionSource=external  InitialConditionForIntegrator=0  InitialConditionForFilter=0  DifferentiatorICPrevScaledInput=0  ExternalReset=level  TrackingMode=off  Kt=1  LimitOutput=on  SatLimitsSource=internal  UpperSaturationLimit=1  LowerSaturationLimit=-1  LinearizeAsGain=on  AntiWindupMode=clamping  Kb=1  LimitIntegrator=off  UpperIntegratorSaturationLimit=inf  LowerIntegratorSaturationLimit=-inf  RndMeth=Simplest  POutMin=[]  POutMax=[]  IOutMin=[]  IOutMax=[]  DOutMin=[]  DOutMax=[]  NOutMin=[]  NOutMax=[]  SumOutMin=[]  SumOutMax=[]  SaturationOutDataTypeStr=Inherit: Inherit via back propagation  SaturationOutMin=[]  SaturationOutMax=[]  PParamMin=[]  PParamMax=[]  IParamMin=[]  IParamMax=[]  DParamMin=[]  DParamMax=[]  NParamMin=[]  NParamMax=[]  KbParamMin=[]  KbParamMax=[]  KtParamMin=[]  KtParamMax=[]  KbOutMin=[]  KbOutMax=[]  KtOutMin=[]  KtOutMax=[]  IntegratorOutMin=[]  IntegratorOutMax=[]  FilterOutMin=[]  FilterOutMax=[]  SumI1OutMin=[]  SumI1OutMax=[]  SumI2OutMin=[]  SumI2OutMax=[]  SumI3OutMin=[]  SumI3OutMax=[]  SumI4OutMin=[]  SumI4OutMax=[]  SumDOutMin=[]  SumDOutMax=[]  DifferentiatorOutMin=[]  DifferentiatorOutMax=[]  FilterDiffOutCoefMin=[]  FilterDiffOutCoefMax=[]  ReciprocalOutMin=[]  ReciprocalOutMax=[]  SumDenOutMin=[]  SumDenOutMax=[]  SumNumOutMin=[]  SumNumOutMax=[]  DivideOutMin=[]  DivideOutMax=[]  UdiffTsProdOutMin=[]  UdiffTsProdOutMax=[]  NTsProdOutMin=[]  NTsProdOutMax=[]  UintegralTsProdOutMin=[]  UintegralTsProdOutMax=[]  UngainTsProdOutMin=[]  UngainTsProdOutMax=[]  ClampingZeroOutDataTypeStr=Inherit: Inherit via back propagation  ClampingZeroOutMin=[]  ClampingZeroOutMax=[]  FilterDenConstantOutDataTypeStr=Inherit: Inherit via back propagation  FilterDenConstantOutMin=[]  FilterDenConstantOutMax=[]  PCopyOutDataTypeStr=Inherit: Inherit via back propagation  PCopyOutMin=[]  PCopyOutMax=[]  NCopyOutDataTypeStr=Inherit: Inherit via back propagation  NCopyOutMin=[]  NCopyOutMax=[]  IntegratorContinuousStateAttributes=''  IntegratorStateMustResolveToSignalObject=off  IntegratorRTWStateStorageClass=Auto  FilterContinuousStateAttributes=''  FilterStateMustResolveToSignalObject=off  FilterRTWStateStorageClass=Auto  ParallelPVariant=ExternalParameters  IdealPVariant=Disabled  IVariant=ExternalParameters  DVariant=Disabled  IntegratorVariant=Discrete  SatVariant=Enabled  AWVariant=DiscClampingParallel  PCopyVariant=Disabled  TRVariant=Disabled  FdbkBlocksVariant=Forward  IdealPFdbkVariant=Disabled  SatFdbkVariant=Disabled  DerivativeFilterVariant=Disabled  NVariant=Disabled  NCopyVariant=Disabled_SignalSpec  FilterICVariant=Disabled  IntegratorICVariant=ExternalICs  ExternalResetVariant=ExternalReset  TRSumVariant=Passthrough  SumFdbkVariant=Disabled  SumVariant=Sum_PI  TsampFilterVariant=InternalTs  TsampNgainVariant=Passthrough  TsampIntegralVariant=Disabled_SignalSpec  ExternalSaturationOutDataTypeStr=Inherit: Same as second input  DerivativeSourceVariant=Disabled  PreIntVariant=InternalPreInt
      settings: LibrarySourceBlock=mcbcontrolslib/PI Controller
  Ki : Constant  Value=Ts * PI_params.Ki_i  OutDataTypeStr=dataType  SampleTime=-1
  Kp : Constant  Value=PI_params.Kp_i  OutDataTypeStr=dataType2  SampleTime=-1
  Logical Operator : Logic  Operator=NOT  IconShape=distinctive  AllPortsSameDT=off  OutDataTypeStr=boolean
  Saturation : Saturate  UpperLimit=0.15  LowerLimit=0.15  RndMeth=Simplest
  Sum : Sum  Inputs=|+-  OutDataTypeStr=Inherit: Same as first input
  Switch : Switch  Criteria=u2 ~= 0  RndMeth=Simplest  SaturateOnIntegerOverflow=off  InputSameDT=off
  Unit Delay : UnitDelay  SampleTime=-1  HasFrameUpgradeWarning=on
  Vd_OpenLoop : DataStoreRead  DataStoreName=Speed_ref  IndexOptions=Index vector (dialog)  Indices=1  OutputSizes=1
  V_ref : Outport  VectorParamsAs1DForOutWhenUnconnected=off
  wires:
  I_ref/1 -> Sum/1
  I_fb/1 -> Sum/2
  Data Store Read2/1 -> Switch/2, Logical Operator/1
  Sum/1 -> Discrete PI Controller with anti-windup & reset/1
  Kp/1 -> Discrete PI Controller with anti-windup & reset/2
  Ki/1 -> Discrete PI Controller with anti-windup & reset/3
  Logical Operator/1 -> Discrete PI Controller with anti-windup & reset/4
  Saturation/1 -> Switch/3
  Switch/1 -> Unit Delay/1, V_ref/1
  Discrete PI Controller with anti-windup & reset/1 -> Switch/1
  Unit Delay/1 -> Discrete PI Controller with anti-windup & reset/5
  Vd_OpenLoop/1 -> Abs/1
  Abs/1 -> Saturation/1

== system mcb_microchip_pmsm_foc_sensorless_dsPIC33EP256MC506/Current Control/Closed Loop Control/Current_Controllers/PI_Controller_Iq ==
  I_ref : Inport
  I_fb : Inport  Port=2
  Data Store Read1 : DataStoreRead  DataStoreName=EnClosedLoop  IndexOptions=Index vector (dialog)  Indices=1  OutputSizes=1
  Discrete PI Controller with anti-windup & reset : slpidlib/PID Controller  Controller=PI  Form=Parallel  TimeDomain=Discrete-time  UseExternalTs=off  SampleTime=-1  IntegratorMethod=Forward Euler  FilterMethod=Forward Euler  ControllerParametersSource=external  P=1  I=1  UseKiTs=on  D=0  UseExternalDerivativeSource=off  N=100  UseFilter=on  TunerSelectOption=Transfer Function Based (PID Tuner App)  InitialConditionSource=external  InitialConditionForIntegrator=0  InitialConditionForFilter=0  DifferentiatorICPrevScaledInput=0  ExternalReset=level  TrackingMode=off  Kt=1  LimitOutput=on  SatLimitsSource=internal  UpperSaturationLimit=1  LowerSaturationLimit=-1  LinearizeAsGain=on  AntiWindupMode=clamping  Kb=1  LimitIntegrator=off  UpperIntegratorSaturationLimit=inf  LowerIntegratorSaturationLimit=-inf  RndMeth=Simplest  POutMin=[]  POutMax=[]  IOutMin=[]  IOutMax=[]  DOutMin=[]  DOutMax=[]  NOutMin=[]  NOutMax=[]  SumOutMin=[]  SumOutMax=[]  SaturationOutDataTypeStr=Inherit: Inherit via back propagation  SaturationOutMin=[]  SaturationOutMax=[]  PParamMin=[]  PParamMax=[]  IParamMin=[]  IParamMax=[]  DParamMin=[]  DParamMax=[]  NParamMin=[]  NParamMax=[]  KbParamMin=[]  KbParamMax=[]  KtParamMin=[]  KtParamMax=[]  KbOutMin=[]  KbOutMax=[]  KtOutMin=[]  KtOutMax=[]  IntegratorOutMin=[]  IntegratorOutMax=[]  FilterOutMin=[]  FilterOutMax=[]  SumI1OutMin=[]  SumI1OutMax=[]  SumI2OutMin=[]  SumI2OutMax=[]  SumI3OutMin=[]  SumI3OutMax=[]  SumI4OutMin=[]  SumI4OutMax=[]  SumDOutMin=[]  SumDOutMax=[]  DifferentiatorOutMin=[]  DifferentiatorOutMax=[]  FilterDiffOutCoefMin=[]  FilterDiffOutCoefMax=[]  ReciprocalOutMin=[]  ReciprocalOutMax=[]  SumDenOutMin=[]  SumDenOutMax=[]  SumNumOutMin=[]  SumNumOutMax=[]  DivideOutMin=[]  DivideOutMax=[]  UdiffTsProdOutMin=[]  UdiffTsProdOutMax=[]  NTsProdOutMin=[]  NTsProdOutMax=[]  UintegralTsProdOutMin=[]  UintegralTsProdOutMax=[]  UngainTsProdOutMin=[]  UngainTsProdOutMax=[]  ClampingZeroOutDataTypeStr=Inherit: Inherit via back propagation  ClampingZeroOutMin=[]  ClampingZeroOutMax=[]  FilterDenConstantOutDataTypeStr=Inherit: Inherit via back propagation  FilterDenConstantOutMin=[]  FilterDenConstantOutMax=[]  PCopyOutDataTypeStr=Inherit: Inherit via back propagation  PCopyOutMin=[]  PCopyOutMax=[]  NCopyOutDataTypeStr=Inherit: Inherit via back propagation  NCopyOutMin=[]  NCopyOutMax=[]  IntegratorContinuousStateAttributes=''  IntegratorStateMustResolveToSignalObject=off  IntegratorRTWStateStorageClass=Auto  FilterContinuousStateAttributes=''  FilterStateMustResolveToSignalObject=off  FilterRTWStateStorageClass=Auto  ParallelPVariant=ExternalParameters  IdealPVariant=Disabled  IVariant=ExternalParameters  DVariant=Disabled  IntegratorVariant=Discrete  SatVariant=Enabled  AWVariant=DiscClampingParallel  PCopyVariant=Disabled  TRVariant=Disabled  FdbkBlocksVariant=Forward  IdealPFdbkVariant=Disabled  SatFdbkVariant=Disabled  DerivativeFilterVariant=Disabled  NVariant=Disabled  NCopyVariant=Disabled_SignalSpec  FilterICVariant=Disabled  IntegratorICVariant=ExternalICs  ExternalResetVariant=ExternalReset  TRSumVariant=Passthrough  SumFdbkVariant=Disabled  SumVariant=Sum_PI  TsampFilterVariant=InternalTs  TsampNgainVariant=Passthrough  TsampIntegralVariant=Disabled_SignalSpec  ExternalSaturationOutDataTypeStr=Inherit: Same as second input  DerivativeSourceVariant=Disabled  PreIntVariant=InternalPreInt
      settings: LibrarySourceBlock=mcbcontrolslib/PI Controller
  Ki : Constant  Value=Ts * PI_params.Ki_i  OutDataTypeStr=dataType  SampleTime=-1
  Kp : Constant  Value=PI_params.Kp_i  OutDataTypeStr=dataType2  SampleTime=-1
  Logical Operator : Logic  Operator=NOT  IconShape=distinctive  AllPortsSameDT=off  OutDataTypeStr=boolean
  Sum : Sum  Inputs=|+-  OutDataTypeStr=Inherit: Same as first input
  Switch : Switch  Criteria=u2 ~= 0  RndMeth=Simplest  SaturateOnIntegerOverflow=off  InputSameDT=off
  Unit Delay : UnitDelay  SampleTime=-1  HasFrameUpgradeWarning=on
  Vq_OpenLoop : Constant  Value=0  OutDataTypeStr=dataType  SampleTime=-1
  V_ref : Outport  VectorParamsAs1DForOutWhenUnconnected=off
  wires:
  I_fb/1 -> Sum/2
  I_ref/1 -> Sum/1
  Kp/1 -> Discrete PI Controller with anti-windup & reset/2
  Sum/1 -> Discrete PI Controller with anti-windup & reset/1
  Ki/1 -> Discrete PI Controller with anti-windup & reset/3
  Logical Operator/1 -> Discrete PI Controller with anti-windup & reset/4
  Data Store Read1/1 -> Switch/2, Logical Operator/1
  Vq_OpenLoop/1 -> Switch/3
  Discrete PI Controller with anti-windup & reset/1 -> Switch/1
  Unit Delay/1 -> Discrete PI Controller with anti-windup & reset/5
  Switch/1 -> Unit Delay/1, V_ref/1

== system mcb_microchip_pmsm_foc_sensorless_dsPIC33EP256MC506/Current Control/Closed Loop Control/Open_Loop_Control/OpentoClosed ==
  Speed_fb : Inport
  Chart : Stateflow chart  TreatAsAtomicUnit=on
  Data Store Read5 : DataStoreRead  DataStoreName=Enable  IndexOptions=Index vector (dialog)  Indices=1  OutputSizes=1
  Data Store Write1 : DataStoreWrite  DataStoreName=EnSpeedCtrl  IndexOptions=Index vector (dialog)  Indices=1  OutputSizes=1
  Data Store Write2 : DataStoreWrite  DataStoreName=EnClosedLoop  IndexOptions=Index vector (dialog)  Indices=1  OutputSizes=1
  Data Type Conversion : DataTypeConversion  OutDataTypeStr=boolean  RndMeth=Simplest  SaturateOnIntegerOverflow=off
  Data Type Conversion1 : DataTypeConversion  SaturateOnIntegerOverflow=off  RndMeth=Floor
  Enable Closed Loop : Constant  OutDataTypeStr=uint16
  Enable Closed Loop1 : Constant  Value=Speed_openLoop_PU*0.8  OutDataTypeStr=dataType
  Open Loop Start-up : Constant  Value=0  OutDataTypeStr=uint16
  Switch2 : Switch  Criteria=u2 > Threshold  Threshold=1  SaturateOnIntegerOverflow=off  InputSameDT=off
  EnClosedLoop : Outport
  wires:
  Open Loop Start-up/1 -> Switch2/3
  Data Store Read5/1 -> Chart/3(En)
  Chart/1(Mode) -> Switch2/2
  Switch2/1 -> Data Type Conversion/1
  Speed_fb/1 -> Chart/2(SpeedFb)
  Enable Closed Loop/1 -> Switch2/1
  Enable Closed Loop1/1 -> Chart/1(Limit)
  Data Type Conversion/1 -> EnClosedLoop/1, Data Store Write2/1
  Chart/2(SpeedCtrl) -> Data Type Conversion1/1
  Data Type Conversion1/1 -> Data Store Write1/1

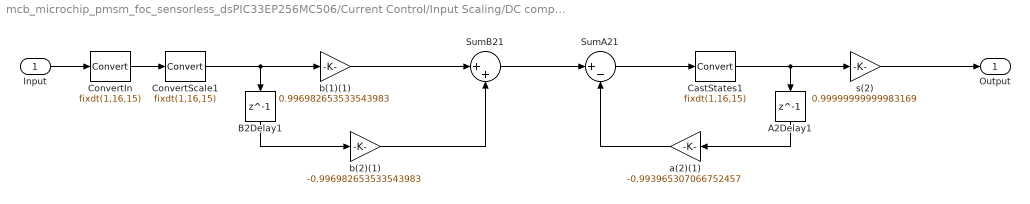
== system mcb_microchip_pmsm_foc_sensorless_dsPIC33EP256MC506/Current Control/Input Scaling/DC component removal/High Pass Filter 1 ==
  Input : Inport
  A2Delay1 : Delay  DelayLength=1  InitialCondition=0
  B2Delay1 : Delay  DelayLength=1  InitialCondition=0
  CastStates1 : DataTypeConversion  OutDataTypeStr=fixdt(1,16,15)
  ConvertIn : DataTypeConversion  OutDataTypeStr=fixdt(1,16,15)  RndMeth=Nearest
  ConvertScale1 : DataTypeConversion  OutDataTypeStr=fixdt(1,16,15)
  SumA21 : Sum  Inputs=|+-  OutDataTypeStr=fixdt(1,32,27)  AccumDataTypeStr=fixdt(1,32,27)  RndMeth=Zero  SaturateOnIntegerOverflow=on
  SumB21 : Sum  Inputs=|++  OutDataTypeStr=fixdt(1,32,28)  AccumDataTypeStr=fixdt(1,32,28)  RndMeth=Zero  SaturateOnIntegerOverflow=on
  a(2)(1) : Gain  Gain=-0.993965307066752457  ParamDataTypeStr=fixdt(1,16,14)  OutDataTypeStr=fixdt(1,32,29)  RndMeth=Zero  SaturateOnIntegerOverflow=on
  b(1)(1) : Gain  Gain=0.996982653533543983  ParamDataTypeStr=fixdt(1,16,15)  OutDataTypeStr=fixdt(1,32,30)  RndMeth=Zero  SaturateOnIntegerOverflow=on
  b(2)(1) : Gain  Gain=-0.996982653533543983  ParamDataTypeStr=fixdt(1,16,15)  OutDataTypeStr=fixdt(1,32,30)  RndMeth=Zero  SaturateOnIntegerOverflow=on
  s(2) : Gain  Gain=0.99999999999983169  ParamDataTypeStr=fixdt(1,16,15)  OutDataTypeStr=fixdt(1,16,11)  RndMeth=Zero  SaturateOnIntegerOverflow=on
  Output : Outport
  wires:
  Input/1 -> ConvertIn/1
  ConvertScale1/1 -> b(1)(1)/1, B2Delay1/1
  b(1)(1)/1 -> SumB21/1
  SumB21/1 -> SumA21/1
  SumA21/1 -> CastStates1/1
  CastStates1/1 -> s(2)/1, A2Delay1/1
  B2Delay1/1 -> b(2)(1)/1
  b(2)(1)/1 -> SumB21/2
  a(2)(1)/1 -> SumA21/2
  A2Delay1/1 -> a(2)(1)/1
  s(2)/1 -> Output/1
  ConvertIn/1 -> ConvertScale1/1

== system mcb_microchip_pmsm_foc_sensorless_dsPIC33EP256MC506/Current Control/Output Scaling/Mode Selector/Subsystem1 ==
  Count : Inport
  Compare To Constant : simulink/Logic and Bit Operations/Compare To Constant  relop=>=  const=1  OutDataTypeStr=boolean
  Compare To Constant1 : simulink/Logic and Bit Operations/Compare To Constant  relop=<  const=1  OutDataTypeStr=boolean
  Data Store Write1 : DataStoreWrite  DataStoreName=EnableFOC  IndexOptions=Index vector (dialog)  Indices=1  OutputSizes=1
  Gain : Gain  Gain=1/(2*PWM_frequency)  OutDataTypeStr=dataType2  RndMeth=Simplest
  Current Offset : Outport
  EnClosedLoop : Outport  Port=2
  tag scope: EnCurOffset=global
  wires:
  Count/1 -> Gain/1
  Gain/1 -> Compare To Constant1/1, Compare To Constant/1
  Compare To Constant/1 -> Data Store Write1/1, EnClosedLoop/1
  Compare To Constant1/1 -> [EnCurOffset], Current Offset/1

== system mcb_microchip_pmsm_foc_sensorless_dsPIC33EP256MC506/Current Control/Output Scaling/Mode Selector/Up Counter ==
  Enable : EnablePort  StatesWhenEnabling=reset
  Add1 : Sum  SaturateOnIntegerOverflow=on
  Constant : Constant  OutDataTypeStr=uint32
  Delay : Delay  DelayLength=1
  Count : Outport  InitialOutput=0
  wires:
  Delay/1 -> Add1/2
  Add1/1 -> Count/1, Delay/1
  Constant/1 -> Add1/1

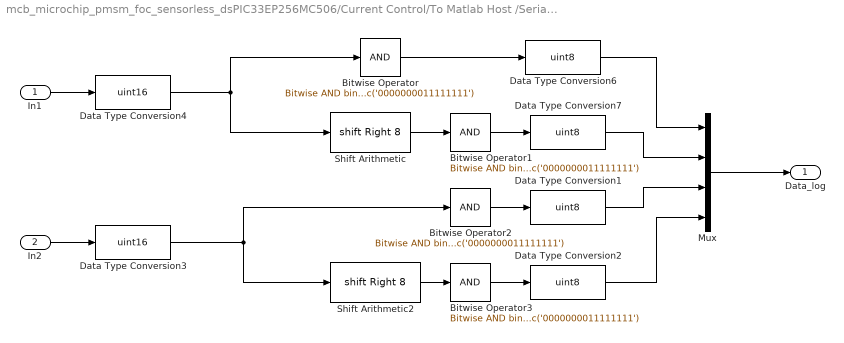
== system mcb_microchip_pmsm_foc_sensorless_dsPIC33EP256MC506/Current Control/To Matlab Host /Serial Send/Debug_Data ==
  In1 : Inport
  In2 : Inport  Port=2
  Bitwise Operator{,1..3} (4 alike) : simulink/Logic and Bit Operations/Bitwise Operator  logicop=AND  UseBitMask=on  BitMask=bin2dec('0000000011111111')  BitMaskRealWorld=Stored Integer
  Data Type Conversion{1..2,6..7} (4 alike) : DataTypeConversion  OutDataTypeStr=uint8  RndMeth=Simplest  SaturateOnIntegerOverflow=off
  Data Type Conversion3 : DataTypeConversion  OutDataTypeStr=uint16  ConvertRealWorld=Stored Integer (SI)  RndMeth=Simplest  SaturateOnIntegerOverflow=off
  Data Type Conversion4 : DataTypeConversion  OutDataTypeStr=uint16  ConvertRealWorld=Stored Integer (SI)  RndMeth=Simplest  SaturateOnIntegerOverflow=off
  Mux : Mux
  Shift Arithmetic : ArithShift  BitShiftNumber=8  BitShiftDirection=Right
  Shift Arithmetic2 : ArithShift  BitShiftNumber=8  BitShiftDirection=Right
  Data_log : Outport
  wires:
  Data Type Conversion3/1 -> Bitwise Operator2/1, Shift Arithmetic2/1
  Bitwise Operator3/1 -> Data Type Conversion2/1
  Shift Arithmetic2/1 -> Bitwise Operator3/1
  Bitwise Operator1/1 -> Data Type Conversion7/1
  Data Type Conversion2/1 -> Mux/4
  Shift Arithmetic/1 -> Bitwise Operator1/1
  Bitwise Operator/1 -> Data Type Conversion6/1
  Data Type Conversion1/1 -> Mux/3
  Bitwise Operator2/1 -> Data Type Conversion1/1
  Data Type Conversion7/1 -> Mux/2
  Data Type Conversion6/1 -> Mux/1
  Data Type Conversion4/1 -> Shift Arithmetic/1, Bitwise Operator/1
  In1/1 -> Data Type Conversion4/1
  In2/1 -> Data Type Conversion3/1
  Mux/1 -> Data_log/1

== system mcb_microchip_pmsm_foc_sensorless_dsPIC33EP256MC506/Current Control/To Matlab Host /Serial Send/SCI_Tx ==
  note: Fast Serial Data Monitoring (32-bit)
  Data_Log : Inport
  Counter Limited : simulink/Sources/Counter Limited  uplimit=599  tsamp=-1
  Data : Subsystem  TreatAsAtomicUnit=on
  End : Subsystem  TreatAsAtomicUnit=on
  If : If  IfExpression=u1 == 0  ElseIfExpressions=u1 == 599
  Start : Subsystem  TreatAsAtomicUnit=on
  wires:
  If/3 -> Data/Action
  Counter Limited/1 -> If/1
  If/2 -> End/Action
  If/1 -> Start/Action
  Data_Log/1 -> End/1(Data), Start/1(Data), Data/1(Data)

== system mcb_microchip_pmsm_foc_sensorless_dsPIC33EP256MC506/Current Control/To Matlab Host /Serial Send/SCI_Tx/Data ==
  Data : Inport
  Action Port : ActionPort  ActionPortLabel=else
  UART Tx : MCHP_Blockset/BUS UART/UART Tx  UART_REF=2  ORDERING=None  AllOrNothing=off  SampleTime=-1  MCHP_MASTERLINK=mcb_microchip_pmsm_foc_sensorless_dsPIC33EP256MC506/Hardware Init/Microchip Master  NSend_Input=off  UART_String=off  NSend_Output=off
      settings: SourceProductName=MPLAB Device Blocks for Simulink
  wires:
  Data/1 -> UART Tx/1

== system mcb_microchip_pmsm_foc_sensorless_dsPIC33EP256MC506/Current Control/To Matlab Host /Serial Send/SCI_Tx/End ==
  Data : Inport
  Action Port : ActionPort  ActionPortLabel=elseif(u1 == 599)
  Mux : Mux  Inputs=2
  Start : Constant  Value=hex2dec('45')  OutDataTypeStr=uint8
  UART Tx : MCHP_Blockset/BUS UART/UART Tx  UART_REF=2  ORDERING=None  AllOrNothing=off  SampleTime=-1  MCHP_MASTERLINK=mcb_microchip_pmsm_foc_sensorless_dsPIC33EP256MC506/Hardware Init/Microchip Master  NSend_Input=off  UART_String=off  NSend_Output=off
      settings: SourceProductName=MPLAB Device Blocks for Simulink
  wires:
  Mux/1 -> UART Tx/1
  Data/1 -> Mux/1
  Start/1 -> Mux/2
